simulink model "PolePlacement_control_model_continuous"  (R2016a)
settings: Solver=ode45  StartTime=0.0  StopTime=2  RelTol=1e-3
model workspace: external: MATLAB File C:\Users\Dick\Documents\GitHub\control-system-lab\dick\Matlab\Pendulum simulation\LQR control\par_struct.m (data not in the file)
values from neighbouring files (symbols this model uses):
  G = G_with_torque    [run_PolePlacement_simulation.m]
  h3 = 0.01    [run_PolePlacement_simulation.m]
  K = place(discr_sys.a,discr_sys.b,pole2)    [run_PolePlacement_simulation.m]
  L = place(discr_sys.a',discr_sys.c',observer_poles)'    [run_PolePlacement_simulation.m]
  N = 2*pi/(w*h3*sqrt(1-zeta^2))    [run_PolePlacement_simulation.m]
  x0 = [pi; 0; 0; 0; 0]    [run_PolePlacement_simulation.m]
undefined symbols (not defined in the file or in its folder): g, k_m, L1, par, tau_e, X, Y, Z
libraries: sm_lib x14, nesl_utility x3
settings Model: Creator=Dick  LastModifiedBy=Dick
settings DataIOCC: InitialState=states  SaveFormat=Array

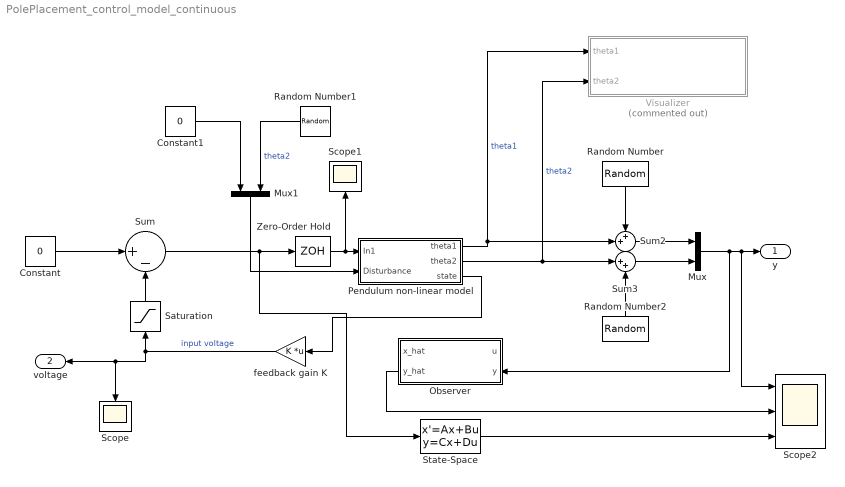
== system PolePlacement_control_model_continuous ==
  Constant : Constant  Value=0  SampleTime=h3
  Constant1 : Constant  Value=0
  Mux : Mux  Inputs=2
  Mux1 : Mux  Inputs=2
  Observer : Subsystem
  Pendulum non-linear model : Subsystem
  Random Number : RandomNumber  Variance=1e-7  SampleTime=h3
  Random Number1 : RandomNumber  Variance=1e-4  SampleTime=h3
  Random Number2 : RandomNumber  Variance=1e-5  SampleTime=h3
  Saturation : Saturate  UpperLimit=1  LowerLimit=-1
  Scope : Scope
  Scope1 : Scope
  Scope2 : Scope  NumInputPorts=3
  State-Space : StateSpace  A=G.a  B=G.b  C=G.c  D=G.d  X0=0
  Sum : Sum  Inputs=|+-
  Sum2 : Sum  Inputs=++|
  Sum3 : Sum  Inputs=|++
  Visualizer : Subsystem  Commented=on
  Zero-Order Hold : ZeroOrderHold  SampleTime=h3
  feedback gain K : Gain  Gain=K  Multiplication=Matrix(K*u)
  y : Outport
  voltage : Outport  Port=2
  wires:
  feedback gain K/1 -> voltage/1, Scope/1, Saturation/1  "input voltage"
  Constant/1 -> Sum/1
  Random Number/1 -> Sum2/1
  Random Number2/1 -> Sum3/2
  Sum3/1 -> Mux/2
  Sum2/1 -> Mux/1
  Mux/1 -> Observer/2(y), Scope2/1, y/1
  Sum/1 -> Zero-Order Hold/1, State-Space/1
  Saturation/1 -> Sum/2
  Constant1/1 -> Mux1/1
  Mux1/1 -> Pendulum non-linear model/2(Disturbance)
  Random Number1/1 -> Mux1/2  "theta2"
  Pendulum non-linear model/2(theta2) -> Visualizer/2(theta2), Sum3/1  "theta2"
  Pendulum non-linear model/1(theta1) -> Sum2/2, Visualizer/1(theta1)  "theta1"
  Zero-Order Hold/1 -> Scope1/1, Pendulum non-linear model/1(In1)
  State-Space/1 -> Scope2/3
  Observer/2(y_hat) -> Scope2/2
  Pendulum non-linear model/3(state) -> feedback gain K/1

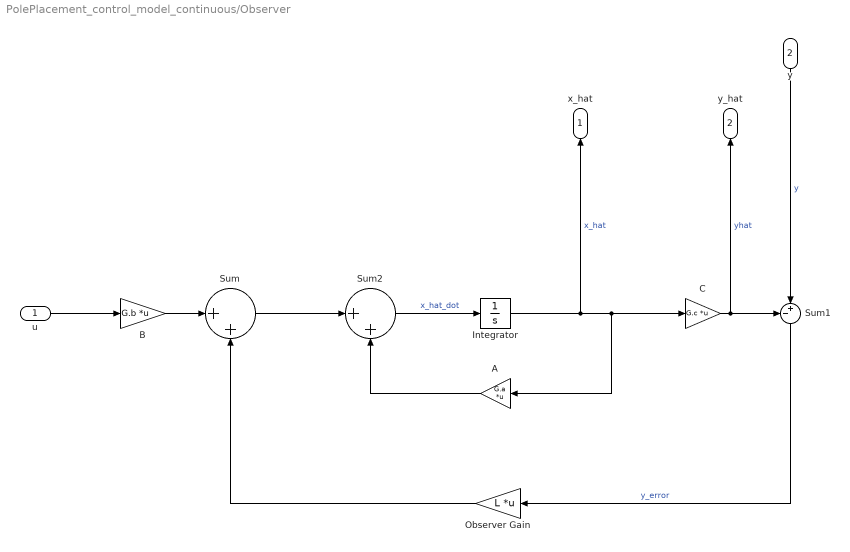
== system PolePlacement_control_model_continuous/Observer ==
  u : Inport
  y : Inport  Port=2
  A : Gain  Gain=G.a  Multiplication=Matrix(K*u)
  B : Gain  Gain=G.b  Multiplication=Matrix(K*u)
  C : Gain  Gain=G.c  Multiplication=Matrix(K*u)
  Integrator : Integrator  InitialCondition=x0
  Observer Gain : Gain  Gain=L  Multiplication=Matrix(K*u)
  Sum : Sum  Inputs=|++
  Sum1 : Sum  Inputs=-+|
  Sum2 : Sum  Inputs=|++
  x_hat : Outport
  y_hat : Outport  Port=2
  wires:
  Observer Gain/1 -> Sum/2
  u/1 -> B/1
  B/1 -> Sum/1
  Sum/1 -> Sum2/1
  Sum2/1 -> Integrator/1  "x_hat_dot"
  Integrator/1 -> x_hat/1, C/1, A/1  "x_hat"
  A/1 -> Sum2/2
  C/1 -> Sum1/1, y_hat/1  "yhat"
  Sum1/1 -> Observer Gain/1  "y_error"
  y/1 -> Sum1/2  "y"

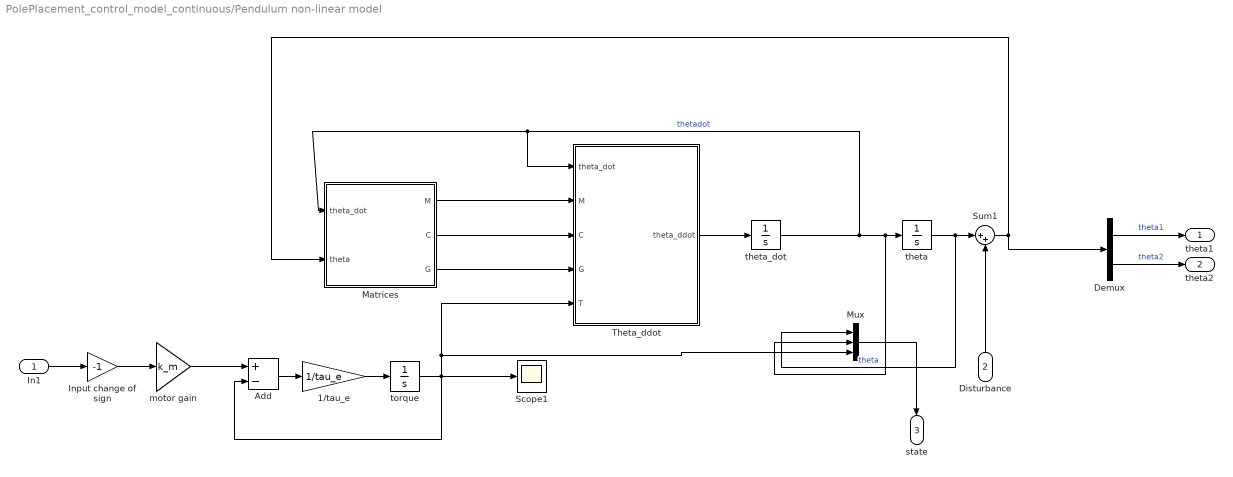
== system PolePlacement_control_model_continuous/Pendulum non-linear model ==
  In1 : Inport
  Disturbance : Inport  Port=2  PortDimensions=2
  "1/tau_e " : Gain  Gain=1/tau_e
  Add : Sum  Inputs=+-
  Demux : Demux  Outputs=2
  Input change of sign : Gain  Gain=-1
  Matrices : MATLAB Function  TreatAsAtomicUnit=on
  Mux : Mux  Inputs=3
  Scope1 : Scope
  Sum1 : Sum  Inputs=|++
  "Theta_ddot " : MATLAB Function  TreatAsAtomicUnit=on
  "motor gain " : Gain  Gain=k_m
  "theta " : Integrator  InitialCondition=[x0(1) x0(2)]  ContinuousStateAttributes='theta_non_linear'
  "theta_dot " : Integrator  InitialCondition=[x0(3) x0(4)]  ContinuousStateAttributes='thetadot_non_linear'
  torque : Integrator  InitialCondition=x0(5)  ContinuousStateAttributes='torque_non_linear'
  theta1 : Outport
  theta2 : Outport  Port=2
  state : Outport  Port=3
  wires:
  torque/1 -> "Theta_ddot "/5(T), Mux/3, Scope1/1, Add/2
  "1/tau_e "/1 -> torque/1
  Add/1 -> "1/tau_e "/1
  "motor gain "/1 -> Add/1
  "theta_dot "/1 -> Mux/2, "theta "/1, "Theta_ddot "/1(theta_dot), Matrices/1(theta_dot)  "thetadot"
  "Theta_ddot "/1(theta_ddot) -> "theta_dot "/1
  Matrices/3(G) -> "Theta_ddot "/4(G)
  Matrices/2(C) -> "Theta_ddot "/3(C)
  Matrices/1(M) -> "Theta_ddot "/2(M)
  Demux/1 -> theta1/1  "theta1"
  Demux/2 -> theta2/1  "theta2"
  In1/1 -> Input change of sign/1
  Disturbance/1 -> Sum1/2
  "theta "/1 -> Mux/1, Sum1/1  "theta"
  Input change of sign/1 -> "motor gain "/1
  Sum1/1 -> Demux/1, Matrices/2(theta)
  Mux/1 -> state/1

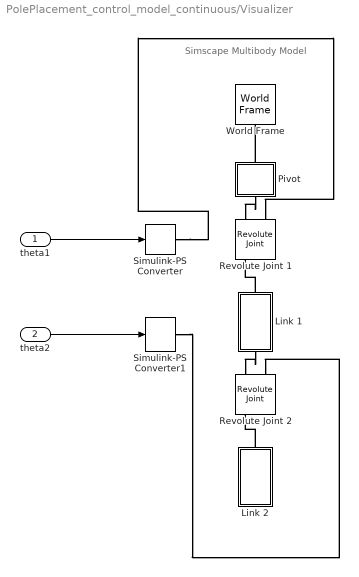
== system PolePlacement_control_model_continuous/Visualizer ==
  note: Simscape Multibody Model
  theta1 : Inport
  theta2 : Inport  Port=2
  Link 1 : Subsystem  Tag=CustomStyle
  Link 2 : Subsystem  Tag=CustomStyle
  Pivot : Subsystem  Tag=CustomStyle
  Revolute Joint 1 : sm_lib/Joints/Revolute Joint  SenseConstraintForce=off  SenseConstraintForceX=off  SenseConstraintForceY=off  SenseConstraintForceZ=off  SenseConstraintTorque=off  SenseConstraintTorqueX=off  SenseConstraintTorqueY=off  SenseConstraintTorqueZ=off  SenseTotalForce=off  SenseTotalForceX=off  SenseTotalForceY=off  SenseTotalForceZ=off  SenseTotalTorque=off  SenseTotalTorqueX=off  SenseTotalTorqueY=off  SenseTotalTorqueZ=off  CompositeWrenchDir=FollowerOnBase  CompositeWrenchFrame=BaseFrame  EquilibriumPosition=0  EquilibriumPositionUnits=rad  SpringStiffness=0  SpringStiffnessUnits=N*m/rad  DampingCoefficient=0  DampingCoefficientUnits=N*m/(rad/s)  TorqueActuationMode=ComputedTorque  MotionActuationMode=InputMotion  SensePosition=on  SenseVelocity=off  SenseAcceleration=off  SenseTorqueForce=off  PositionTargetSpecify=off  PositionTargetPriority=High  PositionTargetValue=0  PositionTargetValueUnits=deg  VelocityTargetSpecify=off  VelocityTargetPriority=High  VelocityTargetValue=0  VelocityTargetValueUnits=rad/s
  Revolute Joint 2 : sm_lib/Joints/Revolute Joint  SenseConstraintForce=off  SenseConstraintForceX=off  SenseConstraintForceY=off  SenseConstraintForceZ=off  SenseConstraintTorque=off  SenseConstraintTorqueX=off  SenseConstraintTorqueY=off  SenseConstraintTorqueZ=off  SenseTotalForce=off  SenseTotalForceX=off  SenseTotalForceY=off  SenseTotalForceZ=off  SenseTotalTorque=off  SenseTotalTorqueX=off  SenseTotalTorqueY=off  SenseTotalTorqueZ=off  CompositeWrenchDir=FollowerOnBase  CompositeWrenchFrame=BaseFrame  EquilibriumPosition=0  EquilibriumPositionUnits=rad  SpringStiffness=0  SpringStiffnessUnits=N*m/rad  DampingCoefficient=0  DampingCoefficientUnits=N*m/(rad/s)  TorqueActuationMode=ComputedTorque  MotionActuationMode=InputMotion  SensePosition=on  SenseVelocity=off  SenseAcceleration=off  SenseTorqueForce=off  PositionTargetSpecify=off  PositionTargetPriority=High  PositionTargetValue=0  PositionTargetValueUnits=deg  VelocityTargetSpecify=off  VelocityTargetPriority=High  VelocityTargetValue=0  VelocityTargetValueUnits=rad/s
  Simulink-PS Converter : nesl_utility/Simulink-PS Converter  PhysicalDomain=network_engine_domain  SubClassName=ps_input  LeftPortType=input  RightPortType=output  PseudoPeriodic=off  Frequencies=[]  NoiseDistribution=none  NoiseParameters=[]  Unit=rad  AffineConversion=off  InputFiltering=on  SimscapeFilterOrder=2  InputFilterTimeConstant=0.001  UdotUserProvided=1
  Simulink-PS Converter1 : nesl_utility/Simulink-PS Converter  PhysicalDomain=network_engine_domain  SubClassName=ps_input  LeftPortType=input  RightPortType=output  PseudoPeriodic=off  Frequencies=[]  NoiseDistribution=none  NoiseParameters=[]  Unit=rad  AffineConversion=off  InputFiltering=on  SimscapeFilterOrder=2  InputFilterTimeConstant=0.001  UdotUserProvided=2
  World Frame : sm_lib/Frames and Transforms/World Frame
  wires:
  theta1/1 -> Simulink-PS Converter/1
  theta2/1 -> Simulink-PS Converter1/1
  connections:
  Link 1/RConn1 -- Revolute Joint 1/RConn1
  Pivot/LConn1 -- World Frame/RConn1
  Link 1/LConn1 -- Revolute Joint 2/LConn1
  Simulink-PS Converter/RConn1 -- Revolute Joint 1/LConn2
  Pivot/RConn1 -- Revolute Joint 1/LConn1
  Simulink-PS Converter1/RConn1 -- Revolute Joint 2/LConn2
  Link 2/RConn1 -- Revolute Joint 2/RConn1

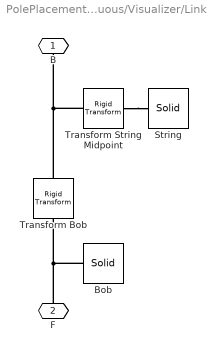
== system PolePlacement_control_model_continuous/Visualizer/Link 1 ==
  Bob : sm_lib/Body Elements/Solid  InertiaType=PointMass  Mass=0  MassUnits=kg  CenterOfMass=[0 0 0]  CenterOfMassUnits=m  MomentsOfInertia=[1 1 1]*1e-3  MomentsOfInertiaUnits=kg*m^2  ProductsOfInertia=[0 0 0]  ProductsOfInertiaUnits=kg*m^2  DensityBased=on  Density=1000  DensityUnits=kg/(m^3)  DoExposeReferenceFrame=on  SerializedFrames=<Frames/>  GraphicType=FromGeometry  MarkerShape=Sphere  MarkerSize=10  MarkerSizeUnits=m  GraphicVisPropType=SimpleVisualProperties  GraphicDiffuseColor=[1.0 0.2 0.0]  GraphicSpecularColor=[0.5 0.5 0.5 1.0]  GraphicAmbientColor=[0.15 0.15 0.15 1.0]  GraphicEmissiveColor=[0.0 0.0 0.0 1.0]  GraphicShininess=75  GraphicOpacity=1.0  GeometryShape=Sphere  RectangleSize=[1 1]  RectangleSizeUnits=m  BrickDimensions=[1 0.1 0.1]  BrickDimensionUnits=m  CylinderRadius=0.1  CylinderRadiusUnits=m  CylinderLength=1  CylinderLengthUnits=m  SphereRadius=0.1  SphereRadiusUnits=m  EllipsoidRadii=[1 1 1]  EllipsoidRadiiUnits=m  ExtrusionCrossSection=[1 1; -1 1; -1 -1; 1 -1]  ExtrusionCrossSectionUnits=m  ExtrusionLength=1  ExtrusionLengthUnits=m  PolygonNumSides=3  PolygonOuterRadius=1  PolygonOuterRadiusUnits=m  ExtGeomFileType=STL  ExtGeomFileUnits=m  RevolutionCrossSection=[1 1; 1 -1; 2 -1; 2 1]  RevolutionCrossSectionUnits=m  RevolutionExtent=Full  RevolutionAngle=180  RevolutionAngleUnits=deg
  String : sm_lib/Body Elements/Solid  InertiaType=CalculateFromGeometry  Mass=0  MassUnits=kg  CenterOfMass=[0 0 0]  CenterOfMassUnits=m  MomentsOfInertia=[1 1 1]*1e-3  MomentsOfInertiaUnits=kg*m^2  ProductsOfInertia=[0 0 0]  ProductsOfInertiaUnits=kg*m^2  DensityBased=on  Density=0  DensityUnits=kg/(m^3)  DoExposeReferenceFrame=on  SerializedFrames=<Frames/>  GraphicType=FromGeometry  MarkerShape=Sphere  MarkerSize=10  MarkerSizeUnits=m  GraphicVisPropType=SimpleVisualProperties  GraphicDiffuseColor=[1.0 0.2 0.0]  GraphicSpecularColor=[0.5 0.5 0.5 1.0]  GraphicAmbientColor=[0.15 0.15 0.15 1.0]  GraphicEmissiveColor=[0.0 0.0 0.0 1.0]  GraphicShininess=75  GraphicOpacity=1.0  GeometryShape=Brick  RectangleSize=[1 1]  RectangleSizeUnits=m  BrickDimensions=[0.01 par.L1 0.01]  BrickDimensionUnits=m  CylinderRadius=0.1  CylinderRadiusUnits=m  CylinderLength=1  CylinderLengthUnits=m  SphereRadius=0.1  SphereRadiusUnits=m  EllipsoidRadii=[1 1 1]  EllipsoidRadiiUnits=m  ExtrusionCrossSection=[1 1; -1 1; -1 -1; 1 -1]  ExtrusionCrossSectionUnits=m  ExtrusionLength=1  ExtrusionLengthUnits=m  PolygonNumSides=3  PolygonOuterRadius=1  PolygonOuterRadiusUnits=m  ExtGeomFileType=STL  ExtGeomFileUnits=m  RevolutionCrossSection=[1 1; 1 -1; 2 -1; 2 1]  RevolutionCrossSectionUnits=m  RevolutionExtent=Full  RevolutionAngle=180  RevolutionAngleUnits=deg
  "Transform Bob " : sm_lib/Frames and Transforms/Rigid Transform  TranslationMethod=StandardAxis  TranslationLengthUnit=m  TranslationStandardAxis=-Y  TranslationStandardOffset=par.L1  TranslationCartesianOffset=[0 0 0]  TranslationROffset=0  TranslationROffsetUnits=m  TranslationZOffset=0  TranslationZOffsetUnits=m  TranslationThetaOffset=0  TranslationThetaOffsetUnits=deg  RotationMethod=None  RotationAngleUnits=deg  RotationStandardAxis=+Z  RotationAngle=0  RotationArbitraryAxis=[0 0 1]  FollAlignAxisA=+X  BaseAlignAxisA=+Y  FollAlignAxisB=+Y  BaseAlignAxisB=+Z  RotationSequenceAxes=FollowerAxes  RotationSequence=XYX  RotationSequenceAngles=[0 0 0]  RotationSequenceAnglesUnits=deg  RotationMatrix=[1 0 0; 0 1 0; 0 0 1]
  Transform String Midpoint : sm_lib/Frames and Transforms/Rigid Transform  TranslationMethod=StandardAxis  TranslationLengthUnit=m  TranslationStandardAxis=-Y  TranslationStandardOffset=par.L1/2  TranslationCartesianOffset=[0 0 0]  TranslationROffset=0  TranslationROffsetUnits=m  TranslationZOffset=0  TranslationZOffsetUnits=m  TranslationThetaOffset=0  TranslationThetaOffsetUnits=deg  RotationMethod=None  RotationAngleUnits=deg  RotationStandardAxis=+Z  RotationAngle=0  RotationArbitraryAxis=[0 0 1]  FollAlignAxisA=+X  BaseAlignAxisA=+Y  FollAlignAxisB=+Y  BaseAlignAxisB=+Z  RotationSequenceAxes=FollowerAxes  RotationSequence=XYX  RotationSequenceAngles=[0 0 0]  RotationSequenceAnglesUnits=deg  RotationMatrix=[1 0 0; 0 1 0; 0 0 1]
  B : PMIOPort  Port=1  Side=Right
  F : PMIOPort  Port=2  Side=Left
  connections:
  "Transform Bob "/LConn1 -- Transform String Midpoint/LConn1 -- B/RConn1
  Bob/RConn1 -- F/RConn1 -- "Transform Bob "/RConn1
  Transform String Midpoint/RConn1 -- String/RConn1

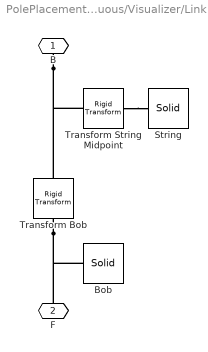
== system PolePlacement_control_model_continuous/Visualizer/Link 2 ==
  Bob : sm_lib/Body Elements/Solid  InertiaType=PointMass  Mass=0  MassUnits=kg  CenterOfMass=[0 0 0]  CenterOfMassUnits=m  MomentsOfInertia=[1 1 1]*1e-3  MomentsOfInertiaUnits=kg*m^2  ProductsOfInertia=[0 0 0]  ProductsOfInertiaUnits=kg*m^2  DensityBased=on  Density=1000  DensityUnits=kg/(m^3)  DoExposeReferenceFrame=on  SerializedFrames=<Frames/>  GraphicType=FromGeometry  MarkerShape=Sphere  MarkerSize=10  MarkerSizeUnits=m  GraphicVisPropType=SimpleVisualProperties  GraphicDiffuseColor=[1.0 0.2 0.0]  GraphicSpecularColor=[0.5 0.5 0.5 1.0]  GraphicAmbientColor=[0.15 0.15 0.15 1.0]  GraphicEmissiveColor=[0.0 0.0 0.0 1.0]  GraphicShininess=75  GraphicOpacity=1.0  GeometryShape=Sphere  RectangleSize=[1 1]  RectangleSizeUnits=m  BrickDimensions=[1 0.1 0.1]  BrickDimensionUnits=m  CylinderRadius=0.1  CylinderRadiusUnits=m  CylinderLength=1  CylinderLengthUnits=m  SphereRadius=0.1  SphereRadiusUnits=m  EllipsoidRadii=[1 1 1]  EllipsoidRadiiUnits=m  ExtrusionCrossSection=[1 1; -1 1; -1 -1; 1 -1]  ExtrusionCrossSectionUnits=m  ExtrusionLength=1  ExtrusionLengthUnits=m  PolygonNumSides=3  PolygonOuterRadius=1  PolygonOuterRadiusUnits=m  ExtGeomFileType=STL  ExtGeomFileUnits=m  RevolutionCrossSection=[1 1; 1 -1; 2 -1; 2 1]  RevolutionCrossSectionUnits=m  RevolutionExtent=Full  RevolutionAngle=180  RevolutionAngleUnits=deg
  String : sm_lib/Body Elements/Solid  InertiaType=CalculateFromGeometry  Mass=0  MassUnits=kg  CenterOfMass=[0 0 0]  CenterOfMassUnits=m  MomentsOfInertia=[1 1 1]*1e-3  MomentsOfInertiaUnits=kg*m^2  ProductsOfInertia=[0 0 0]  ProductsOfInertiaUnits=kg*m^2  DensityBased=on  Density=0  DensityUnits=kg/(m^3)  DoExposeReferenceFrame=on  SerializedFrames=<Frames/>  GraphicType=FromGeometry  MarkerShape=Sphere  MarkerSize=10  MarkerSizeUnits=m  GraphicVisPropType=SimpleVisualProperties  GraphicDiffuseColor=[1.0 0.2 0.0]  GraphicSpecularColor=[0.5 0.5 0.5 1.0]  GraphicAmbientColor=[0.15 0.15 0.15 1.0]  GraphicEmissiveColor=[0.0 0.0 0.0 1.0]  GraphicShininess=75  GraphicOpacity=1.0  GeometryShape=Brick  RectangleSize=[1 1]  RectangleSizeUnits=m  BrickDimensions=[0.01 par.L2 0.01]  BrickDimensionUnits=m  CylinderRadius=0.1  CylinderRadiusUnits=m  CylinderLength=1  CylinderLengthUnits=m  SphereRadius=0.1  SphereRadiusUnits=m  EllipsoidRadii=[1 1 1]  EllipsoidRadiiUnits=m  ExtrusionCrossSection=[1 1; -1 1; -1 -1; 1 -1]  ExtrusionCrossSectionUnits=m  ExtrusionLength=1  ExtrusionLengthUnits=m  PolygonNumSides=3  PolygonOuterRadius=1  PolygonOuterRadiusUnits=m  ExtGeomFileType=STL  ExtGeomFileUnits=m  RevolutionCrossSection=[1 1; 1 -1; 2 -1; 2 1]  RevolutionCrossSectionUnits=m  RevolutionExtent=Full  RevolutionAngle=180  RevolutionAngleUnits=deg
  "Transform Bob " : sm_lib/Frames and Transforms/Rigid Transform  TranslationMethod=StandardAxis  TranslationLengthUnit=m  TranslationStandardAxis=-Y  TranslationStandardOffset=par.L2  TranslationCartesianOffset=[0 0 0]  TranslationROffset=0  TranslationROffsetUnits=m  TranslationZOffset=0  TranslationZOffsetUnits=m  TranslationThetaOffset=0  TranslationThetaOffsetUnits=deg  RotationMethod=None  RotationAngleUnits=deg  RotationStandardAxis=+Z  RotationAngle=0  RotationArbitraryAxis=[0 0 1]  FollAlignAxisA=+X  BaseAlignAxisA=+Y  FollAlignAxisB=+Y  BaseAlignAxisB=+Z  RotationSequenceAxes=FollowerAxes  RotationSequence=XYX  RotationSequenceAngles=[0 0 0]  RotationSequenceAnglesUnits=deg  RotationMatrix=[1 0 0; 0 1 0; 0 0 1]
  Transform String Midpoint : sm_lib/Frames and Transforms/Rigid Transform  TranslationMethod=StandardAxis  TranslationLengthUnit=m  TranslationStandardAxis=-Y  TranslationStandardOffset=par.L2/2  TranslationCartesianOffset=[0 0 0]  TranslationROffset=0  TranslationROffsetUnits=m  TranslationZOffset=0  TranslationZOffsetUnits=m  TranslationThetaOffset=0  TranslationThetaOffsetUnits=deg  RotationMethod=None  RotationAngleUnits=deg  RotationStandardAxis=+Z  RotationAngle=0  RotationArbitraryAxis=[0 0 1]  FollAlignAxisA=+X  BaseAlignAxisA=+Y  FollAlignAxisB=+Y  BaseAlignAxisB=+Z  RotationSequenceAxes=FollowerAxes  RotationSequence=XYX  RotationSequenceAngles=[0 0 0]  RotationSequenceAnglesUnits=deg  RotationMatrix=[1 0 0; 0 1 0; 0 0 1]
  B : PMIOPort  Port=1  Side=Right
  F : PMIOPort  Port=2  Side=Left
  connections:
  Transform String Midpoint/RConn1 -- String/RConn1
  "Transform Bob "/RConn1 -- F/RConn1 -- Bob/RConn1
  B/RConn1 -- Transform String Midpoint/LConn1 -- "Transform Bob "/LConn1

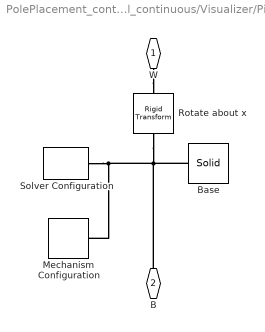
== system PolePlacement_control_model_continuous/Visualizer/Pivot ==
  Base : sm_lib/Body Elements/Solid  InertiaType=PointMass  Mass=0  MassUnits=kg  CenterOfMass=[0 0 0]  CenterOfMassUnits=m  MomentsOfInertia=[1 1 1]*1e-3  MomentsOfInertiaUnits=kg*m^2  ProductsOfInertia=[0 0 0]  ProductsOfInertiaUnits=kg*m^2  DensityBased=on  Density=1000  DensityUnits=kg/(m^3)  DoExposeReferenceFrame=on  SerializedFrames=<Frames/>  GraphicType=FromGeometry  MarkerShape=Sphere  MarkerSize=10  MarkerSizeUnits=m  GraphicVisPropType=SimpleVisualProperties  GraphicDiffuseColor=[0.2 0.2 0.2]  GraphicSpecularColor=[0.5 0.5 0.5 1.0]  GraphicAmbientColor=[0.15 0.15 0.15 1.0]  GraphicEmissiveColor=[0.0 0.0 0.0 1.0]  GraphicShininess=75  GraphicOpacity=1.0  GeometryShape=Cylinder  RectangleSize=[1 1]  RectangleSizeUnits=m  BrickDimensions=[1 0.1 0.1]  BrickDimensionUnits=m  CylinderRadius=0.1  CylinderRadiusUnits=m  CylinderLength=0.1  CylinderLengthUnits=m  SphereRadius=0.1  SphereRadiusUnits=m  EllipsoidRadii=[1 1 1]  EllipsoidRadiiUnits=m  ExtrusionCrossSection=[1 1; -1 1; -1 -1; 1 -1]  ExtrusionCrossSectionUnits=m  ExtrusionLength=1  ExtrusionLengthUnits=m  PolygonNumSides=3  PolygonOuterRadius=1  PolygonOuterRadiusUnits=m  ExtGeomFileType=STL  ExtGeomFileUnits=m  RevolutionCrossSection=[1 1; 1 -1; 2 -1; 2 1]  RevolutionCrossSectionUnits=m  RevolutionExtent=Full  RevolutionAngle=180  RevolutionAngleUnits=deg
  Mechanism Configuration : sm_lib/Utilities/Mechanism Configuration  UniformGravity=Constant  GravityVector=[0 -g 0]  GravityUnits=m/s^2  LinearizationDelta=0.001
  Rotate about x : sm_lib/Frames and Transforms/Rigid Transform  TranslationMethod=StandardAxis  TranslationLengthUnit=m  TranslationStandardAxis=-Y  TranslationStandardOffset=L1/2  TranslationCartesianOffset=[0 0 0]  TranslationROffset=0  TranslationROffsetUnits=m  TranslationZOffset=0  TranslationZOffsetUnits=m  TranslationThetaOffset=0  TranslationThetaOffsetUnits=deg  RotationMethod=StandardAxis  RotationAngleUnits=deg  RotationStandardAxis=+X  RotationAngle=-90  RotationArbitraryAxis=[0 0 1]  FollAlignAxisA=+X  BaseAlignAxisA=+Y  FollAlignAxisB=+Y  BaseAlignAxisB=+Z  RotationSequenceAxes=FollowerAxes  RotationSequence=XYX  RotationSequenceAngles=[0 0 0]  RotationSequenceAnglesUnits=deg  RotationMatrix=[1 0 0; 0 1 0; 0 0 1]
  Solver Configuration : nesl_utility/Solver Configuration  PhysicalDomain=network_engine_domain  SubClassName=solver  LeftPortType=input  RightPortType=generic  Accelerate=off  Tones=[]  Harmonics=[]  SimulateNoise=off  Profile=off  UseLocalSampling=off  EnableSwitchedLinearOptims=on  FrequencyDomain=off  UseCCode=off  RelTol=0.001  AbsTol=1e-06  MinStep=1e-09  ToWorkspace=off  RevertToSquareIcSolve=off  NumHomotopyIterations=100  PhasorMode=off  PhasorModeNumHarmonics=1  OverrideAbsTol=off  DoDC=off  ResidualTolerance=1e-9  UseLocalSolver=off  LocalSolverChoice=NE_BACKWARD_EULER_ADVANCER  LocalSolverSampleTime=.001  DoFixedCost=off  MaxNonlinIter=3  MaxModeIter=2  LinearAlgebra=Sparse  DelaysMemoryBudget=1024  AutomaticFiltering=on  FilteringTimeConstant=0.001
  W : PMIOPort  Port=1  Side=Left
  B : PMIOPort  Port=2  Side=Right
  connections:
  B/RConn1 -- Rotate about x/RConn1 -- Base/RConn1 -- Solver Configuration/RConn1 -- Mechanism Configuration/RConn1
  W/RConn1 -- Rotate about x/LConn1

== matlab function PolePlacement_control_model_continuous/Pendulum non-linear model/Theta_ddot  ==
  data: theta_dot input; M input; C input; G input; theta_ddot output; T input
function theta_ddot = fcn(theta_dot,M,C,G,T)
theta_ddot = [0;0];

theta_ddot = M\[T;0] - M\C*theta_dot - M\G;

== matlab function PolePlacement_control_model_continuous/Pendulum non-linear model/Matrices ==
  data: theta_dot input; theta input; M output; C output; G output
function [M, C, G] = fcn(theta_dot, theta)

M = zeros(2);
C = zeros(2);
G = [0;0];

g = 9.81; 
l1 = 0.1;
l2 = 0.1;
m1 = 0.125;
m2 = 0.05;
c1 = 0.04; % Keeping it negative results in no motion at all, -0.04 or + 0.04?
c2 = 0.06;
I1 = 0.074;
I2 = 0.00012;
b1 = 4.8;
b2 = 0.0002;

P1 = m1*c1^2+m2*l1^2+I1;
P2 = m2*c2^2+ I2;
P3 = m2*l1*c2;
g1 = (m1*c1+m2*l1)*g;
g2 = m2*c2*g;

M = [(P1 + P2 + 2*P3*cos(theta(2)))               (P2 + P3*cos(theta(2))) ;
     (P2 + P3*cos(theta(2)))                       P2                   ];
 
 
C = [(b1 - P3*theta_dot(2)*sin(theta(2)))           (-P3*(theta_dot(1)+theta_dot(2))*sin(theta(2))) ;
     (P3*theta_dot(1)*sin(theta(2)))                 b2                                      ];
     
G = [(-g1*sin(theta(1))-g2*sin(theta(1) + theta(2))) ;
      -g2*sin(theta(1)+theta(2))                   ];
